simulink model "Main"  (Simulink 7.7)
settings: Solver=ode45  StartTime=0.0  StopTime=20.0  RelTol=1e-3
undefined symbols (not defined in the file): sigbuilder_block
settings Model: Creator=FvZ  LastModifiedBy=FvZ

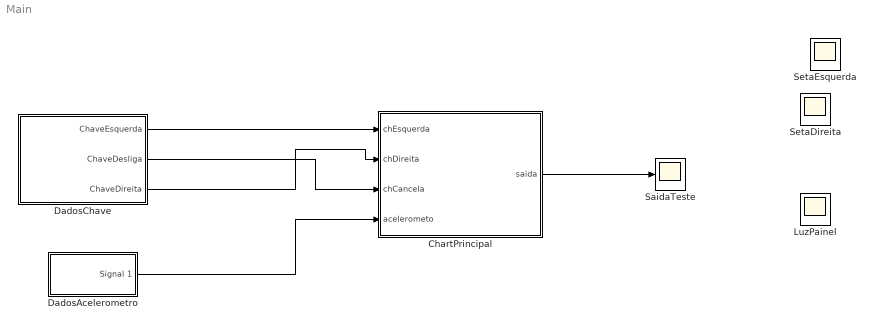
== system Main ==
  ChartPrincipal : Stateflow chart  TreatAsAtomicUnit=on
  DadosAcelerometro : Subsystem  Tag=STV Subsys  LoadFcn=sigbuilder_block('load');  StartFcn=sigbuilder_block('start');  StopFcn=sigbuilder_block('stop');  ClipboardFcn=sigbuilder_block('clipboard');  mask(Sigbuilder block){}
      mask help: Create and generate interchangeable groups of signals whose waveforms are piecewise linear.
      mask init:
      | if ~strcmp(get_param(bdroot(gcbh),'SimulationStatus'),'stopped') tuvar = sigbuilder_block('maskInit'); end
      settings: CopyFcn=sigbuilder_block('copy');  DeleteFcn=sigbuilder_block('delete');  ModelCloseFcn=sigbuilder_block('modelClose');  PreSaveFcn=sigbuilder_block('preSave');  NameChangeFcn=sigbuilder_block('namechange');  OpenFcn=sigbuilder_block('open',[146.25 84 544.5 392.25 ]);  CloseFcn=sigbuilder_block('close');
      mask Display: plot(0, 0, 100, 100,[2, 2, 32, 32, 2], [68, 8, 8, 68, 68],[32, 2], [38, 38], [32, 19, 2],[53, 60, 44], [32, 17, 17, 2],[16, 16, 31, 31]);txt = getActiveGroup(gcbh);text(2, 100, txt,'verticalAlignment', 'top');
  DadosChave : Subsystem  Tag=STV Subsys  LoadFcn=sigbuilder_block('load',[56.25 131.25 550.5 395.25 ]);  StartFcn=sigbuilder_block('start');  StopFcn=sigbuilder_block('stop');  ClipboardFcn=sigbuilder_block('clipboard');  mask(Sigbuilder block){}
      mask help: Create and generate interchangeable groups of signals whose waveforms are piecewise linear.
      mask init:
      | if ~strcmp(get_param(bdroot(gcbh),'SimulationStatus'),'stopped') tuvar = sigbuilder_block('maskInit'); end
      settings: CopyFcn=sigbuilder_block('copy');  DeleteFcn=sigbuilder_block('delete');  ModelCloseFcn=sigbuilder_block('modelClose');  PreSaveFcn=sigbuilder_block('preSave');  NameChangeFcn=sigbuilder_block('namechange');  OpenFcn=sigbuilder_block('open',[403.5 141.75 550.5 395.25 ]);  CloseFcn=sigbuilder_block('close');
      mask Display: plot(0, 0, 100, 100,[2, 2, 32, 32, 2], [68, 8, 8, 68, 68],[32, 2], [38, 38], [32, 19, 2],[53, 60, 44], [32, 17, 17, 2],[16, 16, 31, 31]);txt = getActiveGroup(gcbh);text(2, 100, txt,'verticalAlignment', 'top');
  LuzPainel : Scope
      settings: SaveName=ScopeData2
  SaidaTeste : Scope
      settings: SaveName=ScopeData4
  SetaDireita : Scope
  SetaEsquerda : Scope
  wires:
  DadosChave/1(ChaveEsquerda) -> ChartPrincipal/1(chEsquerda)
  DadosChave/2(ChaveDesliga) -> ChartPrincipal/3(chCancela)
  DadosChave/3(ChaveDireita) -> ChartPrincipal/2(chDireita)
  DadosAcelerometro/1(Signal 1) -> ChartPrincipal/4(acelerometo)
  ChartPrincipal/1(saida) -> SaidaTeste/1

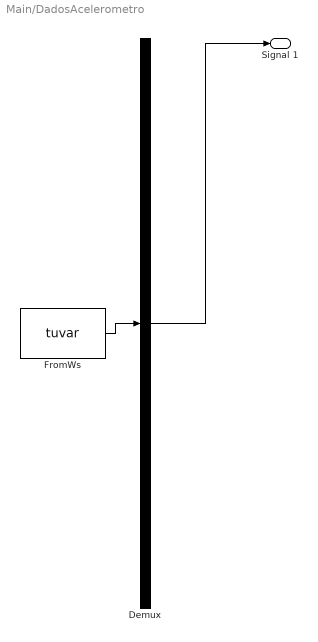
== system Main/DadosAcelerometro ==
  Demux : Demux  Tag=STV Demux  Outputs=1
  FromWs : FromWorkspace  Tag=STV FromWs  VariableName=tuvar  SampleTime=0  SigBuilderData=DataTag0  VnvData=DataTag1
      SigBuilderData=|
      | common.afterFinalStr = 'Extrapolate'
      | common.sampleTime = 0
      | dataSet.timeRange = [0 10]
      | dataSet.name = 'Group 1'
      | sbobj.Groups.Name = 'Group 1'
      | sbobj.Groups.Signals.Name = 'Signal 1'
      | sbobj.Groups.Signals.XData = [0 4 4 6 6 10]
      | sbobj.Groups.Signals.YData = [0 0 1 1 0 0]
  Signal 1 : Outport  Tag=STV Outport
  wires:
  Demux/1 -> Signal 1/1
  FromWs/1 -> Demux/1

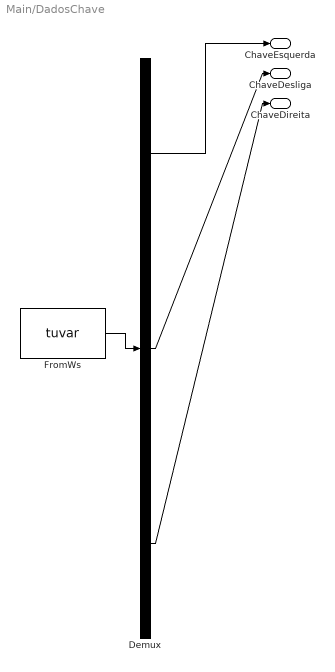
== system Main/DadosChave ==
  Demux : Demux  Tag=STV Demux  Outputs=3
  FromWs : FromWorkspace  Tag=STV FromWs  VariableName=tuvar  SampleTime=0  SigBuilderData=DataTag2  VnvData=DataTag3
      SigBuilderData=|
      | common.afterFinalStr = 'Extrapolate'
      | common.sampleTime = 0
      | dataSet.timeRange = [0 20]
      | dataSet.name = 'Group 1'
      | sbobj.Groups.Name = 'Group 1'
      | sbobj.Groups.Signals(1).Name = 'ChaveEsquerda'
      | sbobj.Groups.Signals(1).XData = [0 4 4 4.42 4.42 5.6 6.02 20]
      | sbobj.Groups.Signals(1).YData = [0 0 1.02 1.02 0 0 0 0]
      | sbobj.Groups.Signals(2).Name = 'ChaveDesliga'
      | sbobj.Groups.Signals(2).XData = [0 5.2 5.28 6.28 6.72 10.2 12.65 12.9 14.15 14.5 20]
      | sbobj.Groups.Signals(2).YData = [0 0 1.04 1 0.02 0 0.02 1 1.02 0 0]
      | sbobj.Groups.Signals(3).Name = 'ChaveDireita'
      | sbobj.Groups.Signals(3).XData = [0 5 7.96 8.08 9.06 9.14 9.84 9.92 10 20]
      | sbobj.Groups.Signals(3).YData = [0 0 0 1.06 1.08 1.08 1.04 0.100465116279 0 0]
      | sbobj.Groups.TimeRange = [0 20]
  ChaveEsquerda : Outport  Tag=STV Outport
  ChaveDesliga : Outport  Tag=STV Outport  Port=2
  ChaveDireita : Outport  Tag=STV Outport  Port=3
  wires:
  Demux/1 -> ChaveEsquerda/1
  FromWs/1 -> Demux/1
  Demux/2 -> ChaveDesliga/1
  Demux/3 -> ChaveDireita/1

== stateflow chart ChartPrincipal ==
  settings: updateMethod=DISCRETE  sampleTime=0.02
  state Desligado
    during: saida=0;
  state Esquerda
    during: saida=2;
  state Direita
    during: saida=1;
  Desligado -> Esquerda [order 1] : [chEsquerda]
  Desligado -> Direita [order 2] : [chDireita]
  Direita -> Desligado : [chCancela]
  (default) -> Desligado
  Esquerda -> Desligado : [chCancela]
  data: chEsquerda input double; chDireita input double; chCancela input double; saida output double; acelerometo input double
